simulink model "UBoot_LowLevelRegler3"  (R2014a)
settings: Solver=ode45  StartTime=0.0  StopTime=5  RelTol=1e-3
libraries: simulink x3
settings Model: Creator=Jonis  LastModifiedBy=Jonis
settings DebuggingCC: UnderspecifiedInitializationDetection=Classic

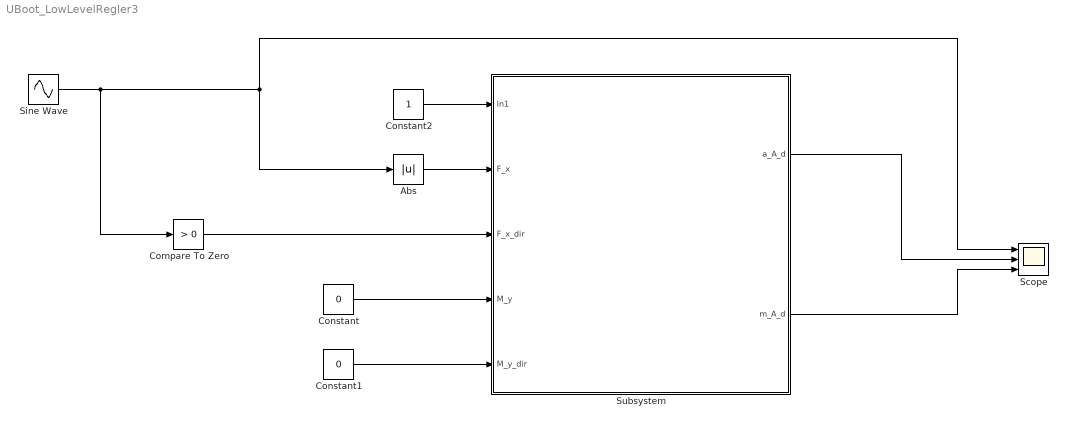
== system UBoot_LowLevelRegler3 ==
  Abs : Abs
  Compare To Zero : simulink/Logic and Bit Operations/Compare To Zero  relop=>  OutDataTypeStr=boolean
  Constant : Constant  Value=0
  Constant1 : Constant  Value=0
  Constant2 : Constant
  Scope : Scope  NumInputPorts=3
      settings: YMin=-5~-5~-5  YMax=5~5~5
  Sine Wave : Sin  Amplitude=100  SampleTime=0
  Subsystem : Subsystem
  wires:
  Sine Wave/1 -> Compare To Zero/1, Abs/1, Scope/1
  Compare To Zero/1 -> Subsystem/3(F_x_dir)
  Constant/1 -> Subsystem/4(M_y)
  Constant1/1 -> Subsystem/5(M_y_dir)
  Subsystem/1(a_A_d) -> Scope/2
  Subsystem/2(m_A_d) -> Scope/3
  Abs/1 -> Subsystem/2(F_x)
  Constant2/1 -> Subsystem/1(In1)

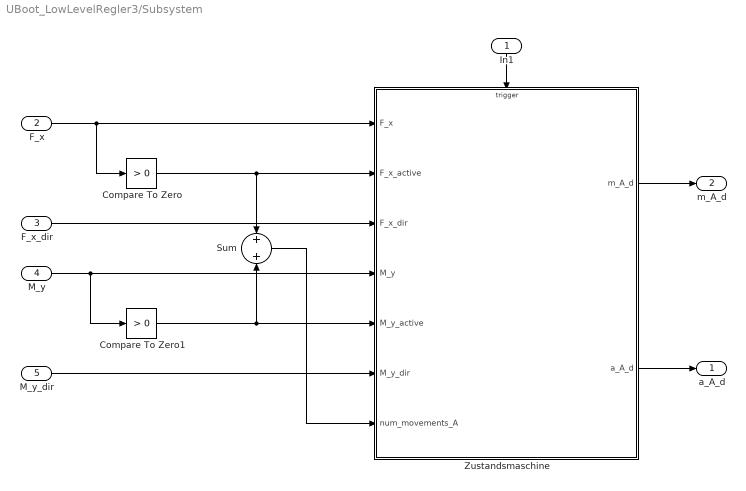
== system UBoot_LowLevelRegler3/Subsystem ==
  In1 : Inport
  F_x : Inport  Port=2
  F_x_dir : Inport  Port=3
  M_y : Inport  Port=4
  M_y_dir : Inport  Port=5
  Compare To Zero : simulink/Logic and Bit Operations/Compare To Zero  relop=>  OutDataTypeStr=boolean
  Compare To Zero1 : simulink/Logic and Bit Operations/Compare To Zero  relop=>  OutDataTypeStr=boolean
  Sum : Sum
  Zustandsmaschine : Stateflow chart  TreatAsAtomicUnit=on
  a_A_d : Outport
  m_A_d : Outport  Port=2
  wires:
  M_y_dir/1 -> Zustandsmaschine/6(M_y_dir)
  Compare To Zero1/1 -> Sum/2, Zustandsmaschine/5(M_y_active)
  Sum/1 -> Zustandsmaschine/7(num_movements_A)
  Zustandsmaschine/2(a_A_d) -> a_A_d/1
  F_x_dir/1 -> Zustandsmaschine/3(F_x_dir)
  Zustandsmaschine/1(m_A_d) -> m_A_d/1
  F_x/1 -> Zustandsmaschine/1(F_x), Compare To Zero/1
  M_y/1 -> Zustandsmaschine/4(M_y), Compare To Zero1/1
  Compare To Zero/1 -> Zustandsmaschine/2(F_x_active), Sum/1
  In1/1 -> Zustandsmaschine/Trigger

== stateflow chart UBoot_LowLevelRegler3/Subsystem/Zustandsmaschine ==
  state one_direction
    state positive_force
      entry: a_A_d = A_angle_positive_force;
      m_A_d = F_x;
    state negative_force
      entry: a_A_d = A_angle_negative_force;
      m_A_d = F_x;
    state positive_torque
      entry: a_A_d = A_angle_positive_torque;
      m_A_d = M_y;
    state negative_torque
      entry: a_A_d = A_angle_negative_torque;
      m_A_d = M_y;
    (junction 23) -> (junction 13)
    (default) -> (junction 13)
    (junction 13) -> positive_force [order 1] : [F_x_active && F_x_dir == 1]
    positive_force -> (junction 23)
    negative_force -> (junction 23)
    (junction 13) -> negative_force [order 2] : [F_x_active && F_x_dir == 0]
    positive_torque -> (junction 23)
    (junction 13) -> negative_torque [order 4] : [M_y_active && M_y_dir == 0]
    (junction 13) -> positive_torque [order 3] : [M_y_active && M_y_dir == 1]
    negative_torque -> (junction 23)
  state no_movement
    entry: a_A_d = 0;
    m_A_d = 0;
  (default) -> no_movement
  no_movement -> one_direction : [num_movements_A > 0]
  one_direction -> no_movement : [num_movements_A < 1]
  data: A_angle_negative_force constant double; A_angle_negative_torque constant double; A_angle_positive_force constant double; A_angle_positive_torque constant double; F_x input; F_x_active input; F_x_dir input; M_y input; M_y_active input; M_y_dir input; num_movements_A input; switch_time constant double; m_A_d output double; a_A_d output double
  events: s input RISING_EDGE_EVENT
